simulink model "mconversionBusWithNegSrcPort"  (Simulink 8.0)
settings: Solver=FixedStepDiscrete  StartTime=0.0  StopTime=10.0  RelTol=1e-3
PreLoadFcn:
  | load myBus.mat
settings Model: Creator=awarlock  LastModifiedBy=htu  ExtModeAutoUpdateStatusClock=off
settings DataIOCC: SignalLoggingSaveFormat=ModelDataLogs
settings OptimizationCC: InitFltsAndDblsToZero=on
settings DebuggingCC: SaveWithParameterizedLinksMsg=none  SignalResolutionControl=TryResolveAllWithWarning  MultiTaskDSMMsg=warning  MultiTaskCondExecSysMsg=none
settings RTWCC: IncludeERTFirstTime=on
settings GRTTargetCC: TargetFcnLib=ansi_tfl_tmw.mat  CombineOutputUpdateFcns=off  GRTInterface=on

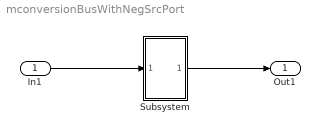
== system mconversionBusWithNegSrcPort ==
  In1 : Inport  OutDataTypeStr=Bus: myBus
  Subsystem : Subsystem  TreatAsAtomicUnit=on
  Out1 : Outport
  wires:
  In1/1 -> Subsystem/1(In1)
  Subsystem/1(Out1) -> Out1/1

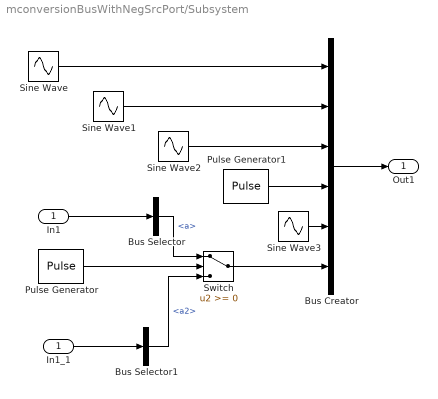
== system mconversionBusWithNegSrcPort/Subsystem ==
  In1 : Inport
  Bus Creator : BusCreator  DialogController=Simulink.DDGSource_Bus  Inputs=6
  Bus Selector : BusSelector  DialogController=Simulink.DDGSource_Bus  OutputSignals=a
  Bus Selector1 : BusSelector  DialogController=Simulink.DDGSource_Bus  OutputSignals=a2
  In1_1 : InportShadow
  Pulse Generator : DiscretePulseGenerator  Period=7  PulseWidth=3  SampleTime=0.1
  Pulse Generator1 : DiscretePulseGenerator  SampleTime=0.1
  Sine Wave{,1..3} (4 alike) : Sin  SampleTime=0.1
  Switch : Switch
  Out1 : Outport
  wires:
  In1/1 -> Bus Selector/1
  In1_1/1 -> Bus Selector1/1
  Bus Selector/1 -> Switch/1  "<a>"
  Pulse Generator/1 -> Switch/2
  Bus Selector1/1 -> Switch/3  "<a2>"
  Bus Creator/1 -> Out1/1
  Switch/1 -> Bus Creator/6
  Sine Wave/1 -> Bus Creator/1
  Sine Wave1/1 -> Bus Creator/2
  Sine Wave2/1 -> Bus Creator/3
  Pulse Generator1/1 -> Bus Creator/4
  Sine Wave3/1 -> Bus Creator/5
